simulink model "state_space_model"  (R2020a)
settings: Solver=VariableStepAuto  StartTime=0.0  StopTime=1000  RelTol=1e-3
settings Model: Creator=啊包PC  LastModifiedBy=啊包PC

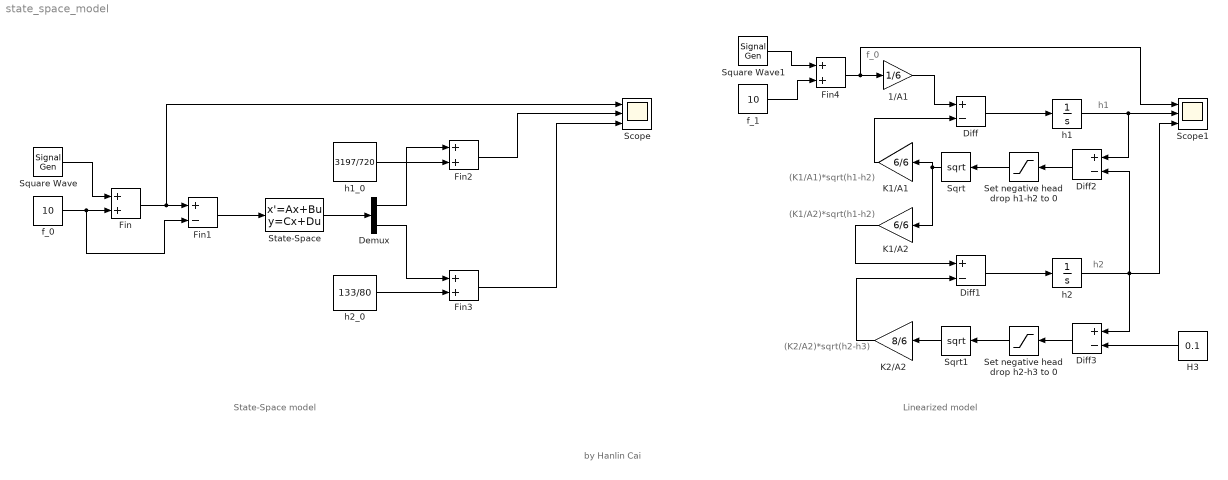
== system state_space_model ==
  note: h1
  note: (K2/A2)*sqrt(h2-h3)
  note: (K1/A1)*sqrt(h1-h2)
  note: h2
  note: f_0
  note: Linearized model
  note: (K1/A2)*sqrt(h1-h2)
  note: State-Space model
  note: by Hanlin Cai
  1/A1 : Gain  Gain=1/6
  Demux : Demux  Outputs=2
  Diff{,1..3} (4 alike) : Sum  Inputs=+-
  Fin{,2..4} (4 alike) : Sum
  Fin1 : Sum  Inputs=+-
  H3 : Constant  Value=0.1
  K1/A1 : Gain  Gain=6/6
  K1/A2 : Gain  Gain=6/6
  K2/A2 : Gain  Gain=8/6
  Scope : Scope  NumInputPorts=3
  Scope1 : Scope  NumInputPorts=3
  Set negative head drop h1-h2 to 0 : Saturate  UpperLimit=Inf  LowerLimit=0  ZeroCross=off
  Set negative head drop h2-h3 to 0 : Saturate  UpperLimit=Inf  LowerLimit=0  ZeroCross=off
  Sqrt : Sqrt  SaturateOnIntegerOverflow=on
  Sqrt1 : Sqrt  SaturateOnIntegerOverflow=on
  Square Wave : SignalGenerator  WaveForm=square  Amplitude=0.3*10  Frequency=1/60
  Square Wave1 : SignalGenerator  WaveForm=square  Amplitude=0.3*10  Frequency=1/60
  State-Space : StateSpace  A="[-0.3 0.3 ; 0.3 -5/6  ]"  B=[1/6 ; 0]  C=[1,0 ; 0 ,1 ]  D=[0 ; 0]  InitialCondition=0
  f_0 : Constant  Value=10
  f_1 : Constant  Value=10
  h1 : Integrator
  h1_0 : Constant  Value=3197/720
  h2 : Integrator
  h2_0 : Constant  Value=133/80
  wires:
  Square Wave/1 -> Fin/1
  f_0/1 -> Fin1/2, Fin/2
  Fin/1 -> Scope/1, Fin1/1
  Fin1/1 -> State-Space/1
  State-Space/1 -> Demux/1
  Fin2/1 -> Scope/2
  Demux/2 -> Fin3/1
  h2_0/1 -> Fin3/2
  Fin3/1 -> Scope/3
  Fin4/1 -> Scope1/1, 1/A1/1
  H3/1 -> Diff3/2
  Set negative head drop h2-h3 to 0/1 -> Sqrt1/1
  Diff2/1 -> Set negative head drop h1-h2 to 0/1
  Diff1/1 -> h2/1
  1/A1/1 -> Diff/1
  Sqrt1/1 -> K2/A2/1
  Square Wave1/1 -> Fin4/1
  Diff3/1 -> Set negative head drop h2-h3 to 0/1
  h2/1 -> Diff3/1, Diff2/2, Scope1/3
  K1/A2/1 -> Diff1/1
  Set negative head drop h1-h2 to 0/1 -> Sqrt/1
  Diff/1 -> h1/1
  Sqrt/1 -> K1/A2/1, K1/A1/1
  f_1/1 -> Fin4/2
  h1/1 -> Scope1/2, Diff2/1
  K2/A2/1 -> Diff1/2
  K1/A1/1 -> Diff/2
  h1_0/1 -> Fin2/2
  Demux/1 -> Fin2/1
